simulink model "New_Traction_Control_4wheel"  (R2016a)
settings: Solver=VariableStepAuto  StartTime=0.0  StopTime=20  RelTol=1e-3
PreLoadFcn:
  | load CarSim_FE4.mat
  | load Vehicle_information_test_0118_2017.mat
libraries: fl_lib x27, nesl_utility x18, sdl_lib x8
settings Model: Creator=Ping  LastModifiedBy=Ping

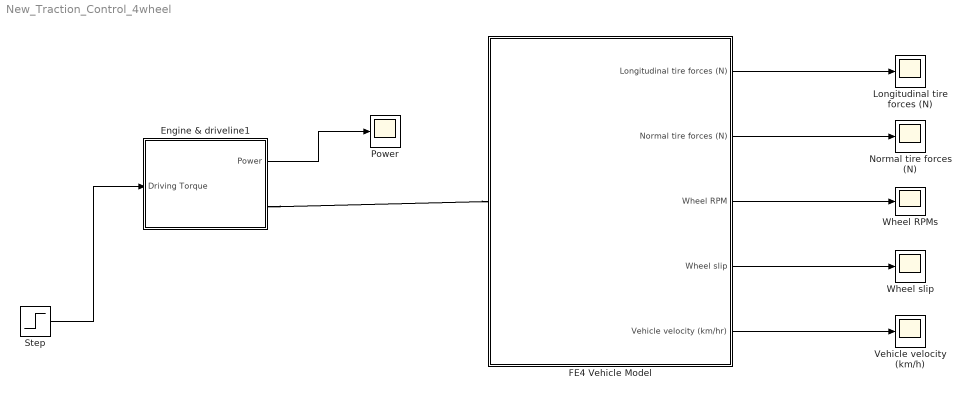
== system New_Traction_Control_4wheel ==
  Engine & driveline1 : Subsystem
  FE4 Vehicle Model : Subsystem
  Longitudinal tire forces (N) : Scope
  Normal tire forces (N) : Scope
  Power : Scope
  Step : Step  Time=10  After=500  SampleTime=0
  Vehicle velocity (km/h) : Scope
  Wheel RPMs : Scope
  Wheel slip : Scope
  wires:
  FE4 Vehicle Model/4(Wheel slip) -> Wheel slip/1
  FE4 Vehicle Model/2(Normal tire forces (N)) -> Normal tire forces (N)/1
  FE4 Vehicle Model/3(Wheel RPM) -> Wheel RPMs/1
  FE4 Vehicle Model/1(Longitudinal tire forces (N)) -> Longitudinal tire forces (N)/1
  FE4 Vehicle Model/5(Vehicle velocity (km/hr)) -> Vehicle velocity (km/h)/1
  Step/1 -> Engine & driveline1/1(Driving Torque)
  Engine & driveline1/1(Power) -> Power/1
  connections:
  Engine & driveline1/RConn1 -- FE4 Vehicle Model/LConn1

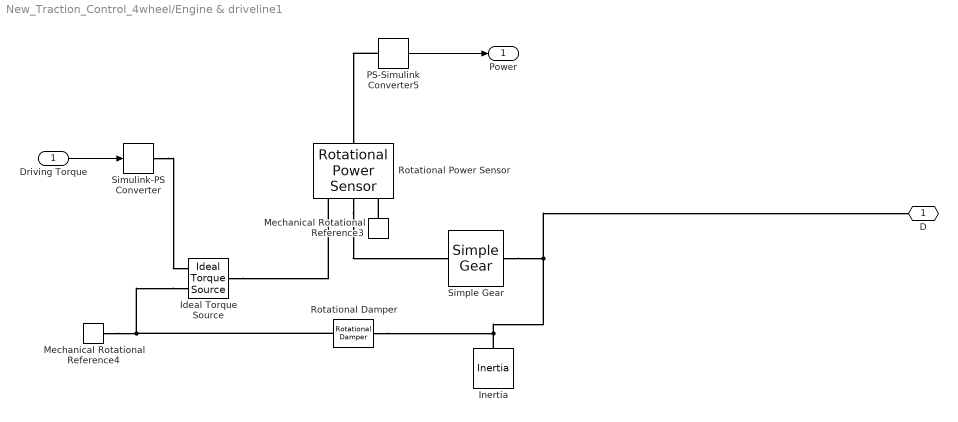
== system New_Traction_Control_4wheel/Engine & driveline1 ==
  Driving Torque : Inport
  Ideal Torque Source : fl_lib/Mechanical/Mechanical Sources/Ideal Torque Source
  Inertia : fl_lib/Mechanical/Rotational Elements/Inertia  inertia=0.015 kg*m^2  w_specify=on  w_priority=Low  w=0 rad/s  t_specify=off  t_priority=Low  t=0 N*m
  Mechanical Rotational Reference3 : fl_lib/Mechanical/Rotational Elements/Mechanical Rotational Reference
  Mechanical Rotational Reference4 : fl_lib/Mechanical/Rotational Elements/Mechanical Rotational Reference
  PS-Simulink Converter5 : nesl_utility/PS-Simulink Converter  PhysicalDomain=network_engine_domain  SubClassName=ps_output  LeftPortType=input  RightPortType=output  PseudoPeriodic=off  Frequencies=[]  Unit=kW  AffineConversion=off
  Rotational Damper : fl_lib/Mechanical/Rotational Elements/Rotational Damper  D=0.001 N*m/(rad/s)  w_specify=off  w_priority=None  w=0 rad/s  t_specify=on  t_priority=Low  t=0 N*m
  Rotational Power Sensor : sdl_lib/Sensors/Rotational Power Sensor  measurement_type=1  averaging_period=1 s  max_speed=1000 rpm  max_frequency=1000 Hz
  Simple Gear : sdl_lib/Gears/Simple Gear  ratio=4.6  rotation_direction=1  friction_model=1  T_noload=0.1 N*m  T_nom=5 N*m  efficiency_nom=0.8  efficiency=0.8  mu_visc=[ 0 0 ] N*m/(rad/s)  w_thr=0.01 rad/s  pwr_thr=0.001 W  temperature_TLU=[ 280 300 320 ] K  load_TLU=[ 1 5 10 ] N*m  efficiency_TLU=[ 0.95 0.9 0.85 ]  efficiency_TLU2=[ 0.85 0.8 0.75; 0.95 0.9 0.85; 0.85 0.8 0.7 ]  thermal_mass=50 J/K  T_init=300 K
  Simulink-PS Converter : nesl_utility/Simulink-PS Converter  PhysicalDomain=network_engine_domain  SubClassName=ps_input  LeftPortType=input  RightPortType=output  PseudoPeriodic=off  Frequencies=[]  NoiseDistribution=none  NoiseParameters=[]  Unit=N*m  AffineConversion=off  InputFiltering=off  SimscapeFilterOrder=1  InputFilterTimeConstant=0.001  UdotUserProvided=1
  D : PMIOPort  Port=1  Side=Right
  Power : Outport
  wires:
  Driving Torque/1 -> Simulink-PS Converter/1
  PS-Simulink Converter5/1 -> Power/1
  connections:
  Simple Gear/RConn1 -- D/RConn1 -- Rotational Damper/RConn1 -- Inertia/LConn1
  Ideal Torque Source/RConn2 -- Mechanical Rotational Reference4/LConn1 -- Rotational Damper/LConn1
  PS-Simulink Converter5/LConn1 -- Rotational Power Sensor/RConn1
  Mechanical Rotational Reference3/LConn1 -- Rotational Power Sensor/LConn3
  Rotational Power Sensor/LConn2 -- Simple Gear/LConn1
  Simulink-PS Converter/RConn1 -- Ideal Torque Source/RConn1
  Ideal Torque Source/LConn1 -- Rotational Power Sensor/LConn1

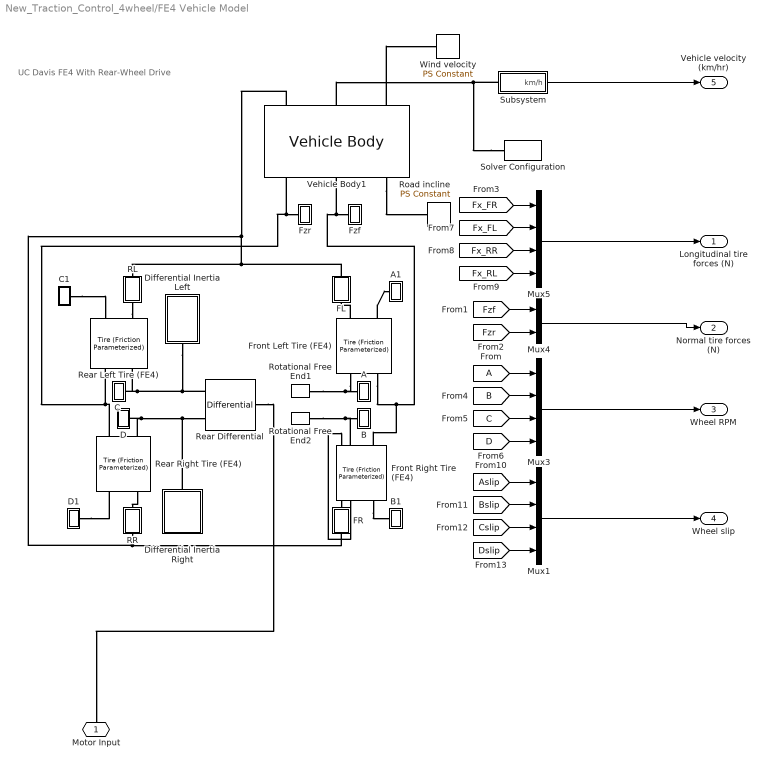
== system New_Traction_Control_4wheel/FE4 Vehicle Model ==
  note: UC Davis FE4 With Rear-Wheel Drive
  A : Subsystem
  A1 : Subsystem
  B : Subsystem
  B1 : Subsystem
  C : Subsystem
  C1 : Subsystem
  D : Subsystem
  D1 : Subsystem
  Differential Inertia Left : Subsystem
  Differential Inertia Right : Subsystem
  FL : Subsystem
  FR : Subsystem
  Front Left Tire (FE4) : sdl_lib/Tires & Vehicles/Tire (Friction Parameterized)  r_tire=r_tire m  mu_static=3  friction_model=2  mu_kinetic=0.7  slip_vector=SL  mu_kinetic_vector=Tire_nu  interp_method=2  extrap_method=1  model_compliance=0  stiffness=1e+6 N/m  damping=1000 N/(m/s)  model_inertia=1  tire_inertia=jt kg*m^2  initial_velocity=0 rad/s  model_resistance=1  resistance_model=1  coeff=0.015  p_tire=250e3 Pa  alpha=-0.003  beta=0.97  coeff_a=84e-4  coeff_b=6.2e-4 s/m  coeff_c=1.6e-4 s^2/m^2  v_thr=1e-3 m/s  v_tol=0.01 m/s  F_min=10 N  initial_traction_state=1
  Front Right Tire (FE4) : sdl_lib/Tires & Vehicles/Tire (Friction Parameterized)  r_tire=r_tire m  mu_static=3  friction_model=2  mu_kinetic=0.7  slip_vector=SL  mu_kinetic_vector=Tire_nu  interp_method=2  extrap_method=1  model_compliance=0  stiffness=1e+6 N/m  damping=1000 N/(m/s)  model_inertia=1  tire_inertia=jt kg*m^2  initial_velocity=0 rad/s  model_resistance=1  resistance_model=1  coeff=0.015  p_tire=250e3 Pa  alpha=-0.003  beta=0.97  coeff_a=84e-4  coeff_b=6.2e-4 s/m  coeff_c=1.6e-4 s^2/m^2  v_thr=1e-3 m/s  v_tol=0.01 m/s  F_min=10 N  initial_traction_state=1
  Fzf : Subsystem
  Fzr : Subsystem
  Mux1 : Mux
  Mux3 : Mux
  Mux4 : Mux  Inputs=2
  Mux5 : Mux
  RL : Subsystem
  RR : Subsystem
  Rear Differential : sdl_lib/Gears/Differential  driveshaft_location=2  cd_ratio=1  friction_model=1  efficiency=[ 0.85 0.92 ]  mu_visc=[ 0 0 ] N*m/(rad/s)  pwr_thr=[ 0.001 0.001 ] W  carrier_inertia=0 kg*m^2  planet_inertia=0 kg*m^2  temperature_TLU=[ 280 300 320 ] K  efficiency_ss_TLU=[ 0.95 0.9 0.85 ]  efficiency_cd_TLU=[ 0.95 0.9 0.85 ]  thermal_mass=50 J/K  T_init=300 K
  Rear Left Tire (FE4) : sdl_lib/Tires & Vehicles/Tire (Friction Parameterized)  r_tire=r_tire m  mu_static=3  friction_model=2  mu_kinetic=0.7  slip_vector=SL  mu_kinetic_vector=Tire_nu  interp_method=2  extrap_method=1  model_compliance=0  stiffness=1e+6 lbf/ft  damping=1000 N/(m/s)  model_inertia=1  tire_inertia=jt kg*m^2  initial_velocity=0 rad/s  model_resistance=1  resistance_model=1  coeff=0.015  p_tire=250e3 Pa  alpha=-0.003  beta=0.97  coeff_a=84e-4  coeff_b=6.2e-4 s/m  coeff_c=1.6e-4 s^2/m^2  v_thr=1e-3 m/s  v_tol=0.01 m/s  F_min=10 N  initial_traction_state=1
  Rear Right Tire (FE4) : sdl_lib/Tires & Vehicles/Tire (Friction Parameterized)  r_tire=r_tire m  mu_static=3  friction_model=2  mu_kinetic=0.7  slip_vector=SL  mu_kinetic_vector=Tire_nu  interp_method=2  extrap_method=1  model_compliance=0  stiffness=1e+6 lbf/ft  damping=1000 N/(m/s)  model_inertia=1  tire_inertia=jt kg*m^2  initial_velocity=0 rad/s  model_resistance=1  resistance_model=1  coeff=0.015  p_tire=250e3 Pa  alpha=-0.003  beta=0.97  coeff_a=84e-4  coeff_b=6.2e-4 s/m  coeff_c=1.6e-4 s^2/m^2  v_thr=1e-3 m/s  v_tol=0.01 m/s  F_min=10 N  initial_traction_state=1
  Road incline : fl_lib/Physical Signals/Sources/PS Constant  constant=0
  Rotational Free End1 : fl_lib/Mechanical/Rotational Elements/Rotational Free End  w_specify=on  w_priority=Low  w=0 rad/s
  Rotational Free End2 : fl_lib/Mechanical/Rotational Elements/Rotational Free End  w_specify=on  w_priority=Low  w=0 rad/s
  Solver Configuration : nesl_utility/Solver Configuration  PhysicalDomain=network_engine_domain  SubClassName=solver  LeftPortType=input  RightPortType=generic  Accelerate=off  Tones=[]  Harmonics=[]  SimulateNoise=off  Profile=off  UseLocalSampling=off  EnableSwitchedLinearOptims=on  FrequencyDomain=off  UseCCode=off  RelTol=0.001  AbsTol=1e-06  MinStep=1e-09  ToWorkspace=off  RevertToSquareIcSolve=off  NumHomotopyIterations=100  PhasorMode=off  PhasorModeNumHarmonics=1  OverrideAbsTol=off  DoDC=off  ResidualTolerance=1e-9  UseLocalSolver=off  LocalSolverChoice=NE_BACKWARD_EULER_ADVANCER  LocalSolverSampleTime=0.1  DoFixedCost=off  MaxNonlinIter=3  MaxModeIter=2  LinearAlgebra=Sparse  DelaysMemoryBudget=1024  AutomaticFiltering=on  FilteringTimeConstant=0.001
  Subsystem : Subsystem
  Vehicle Body1 : sdl_lib/Tires & Vehicles/Vehicle Body  mass=m_total kg  n_w=2  x_f=aa m  x_r=bb m  y_c=hf m  area=frontal_area m^2  Cd=Cd  v0=0 m/s
  Wind velocity : fl_lib/Physical Signals/Sources/PS Constant  constant=0
  Motor Input : PMIOPort  Port=1  Side=Left
  Longitudinal tire forces (N) : Outport
  Normal tire forces (N) : Outport  Port=2
  Wheel RPM : Outport  Port=3
  Wheel slip : Outport  Port=4
  Vehicle velocity (km/hr) : Outport  Port=5
  wires:
  Subsystem/1(km/h) -> Vehicle velocity (km/hr)/1
  [A] -> Mux3/1
  [Fx_FL] -> Mux5/2
  [Fx_FR] -> Mux5/1
  [Fx_RR] -> Mux5/3
  [Fx_RL] -> Mux5/4
  [Aslip] -> Mux1/1
  [Dslip] -> Mux1/4
  Mux1/1 -> Wheel slip/1
  [Bslip] -> Mux1/2
  [Fzr] -> Mux4/2
  Mux4/1 -> Normal tire forces (N)/1
  [Cslip] -> Mux1/3
  [C] -> Mux3/3
  [B] -> Mux3/2
  [D] -> Mux3/4
  Mux3/1 -> Wheel RPM/1
  [Fzf] -> Mux4/1
  Mux5/1 -> Longitudinal tire forces (N)/1
  connections:
  C1/LConn1 -- Rear Left Tire (FE4)/RConn1
  Rear Right Tire (FE4)/RConn2 -- RR/LConn1
  Rotational Free End2/LConn1 -- Front Right Tire (FE4)/LConn2 -- B/LConn1
  A/LConn1 -- Rotational Free End1/LConn1 -- Front Left Tire (FE4)/LConn2
  Rear Differential/LConn1 -- Motor Input/RConn1
  Front Right Tire (FE4)/RConn1 -- B1/LConn1
  Vehicle Body1/LConn3 -- Wind velocity/RConn1
  D1/LConn1 -- Rear Right Tire (FE4)/RConn1
  Front Left Tire (FE4)/RConn1 -- A1/LConn1
  RR/RConn1 -- FR/RConn1 -- Vehicle Body1/LConn1 -- FL/RConn1 -- RL/RConn1
  D/LConn1 -- Rear Right Tire (FE4)/LConn2 -- Differential Inertia Right/RConn1 -- Rear Differential/RConn2
  Fzr/LConn1 -- Rear Right Tire (FE4)/LConn1 -- Rear Left Tire (FE4)/LConn1 -- Vehicle Body1/RConn1
  Solver Configuration/RConn1 -- Vehicle Body1/LConn2 -- Subsystem/LConn1
  Fzf/LConn1 -- Front Left Tire (FE4)/LConn1 -- Front Right Tire (FE4)/LConn1 -- Vehicle Body1/RConn2
  Vehicle Body1/RConn3 -- Road incline/RConn1
  RL/LConn1 -- Rear Left Tire (FE4)/RConn2
  Front Right Tire (FE4)/RConn2 -- FR/LConn1
  Front Left Tire (FE4)/RConn2 -- FL/LConn1
  Rear Differential/RConn1 -- C/LConn1 -- Rear Left Tire (FE4)/LConn2 -- Differential Inertia Left/RConn1

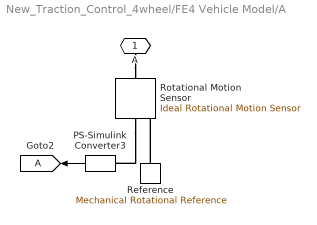
== system New_Traction_Control_4wheel/FE4 Vehicle Model/A ==
  PS-Simulink Converter3 : nesl_utility/PS-Simulink Converter  PhysicalDomain=network_engine_domain  SubClassName=ps_output  LeftPortType=input  RightPortType=output  PseudoPeriodic=off  Frequencies=[]  Unit=rpm  AffineConversion=off
  Reference : fl_lib/Mechanical/Rotational Elements/Mechanical Rotational Reference
  Rotational Motion Sensor : fl_lib/Mechanical/Mechanical Sensors/Ideal Rotational Motion Sensor  offset=0 rad
  A : PMIOPort  Port=1  Side=Left
  tag scope: A=global
  wires:
  PS-Simulink Converter3/1 -> [A]
  connections:
  Rotational Motion Sensor/RConn2 -- PS-Simulink Converter3/LConn1
  Reference/LConn1 -- Rotational Motion Sensor/RConn1
  A/RConn1 -- Rotational Motion Sensor/LConn1

== system New_Traction_Control_4wheel/FE4 Vehicle Model/A1 ==
  PS-Simulink Converter : nesl_utility/PS-Simulink Converter  PhysicalDomain=network_engine_domain  SubClassName=ps_output  LeftPortType=input  RightPortType=output  PseudoPeriodic=off  Frequencies=[]  Unit=1  AffineConversion=off
  S : PMIOPort  Port=1  Side=Left
  tag scope: Aslip=global
  wires:
  PS-Simulink Converter/1 -> [Aslip]
  connections:
  S/RConn1 -- PS-Simulink Converter/LConn1

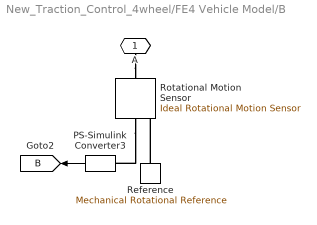
== system New_Traction_Control_4wheel/FE4 Vehicle Model/B ==
  PS-Simulink Converter3 : nesl_utility/PS-Simulink Converter  PhysicalDomain=network_engine_domain  SubClassName=ps_output  LeftPortType=input  RightPortType=output  PseudoPeriodic=off  Frequencies=[]  Unit=rpm  AffineConversion=off
  Reference : fl_lib/Mechanical/Rotational Elements/Mechanical Rotational Reference
  Rotational Motion Sensor : fl_lib/Mechanical/Mechanical Sensors/Ideal Rotational Motion Sensor  offset=0 rad
  A : PMIOPort  Port=1  Side=Left
  tag scope: B=global
  wires:
  PS-Simulink Converter3/1 -> [B]
  connections:
  A/RConn1 -- Rotational Motion Sensor/LConn1
  Reference/LConn1 -- Rotational Motion Sensor/RConn1
  Rotational Motion Sensor/RConn2 -- PS-Simulink Converter3/LConn1

== system New_Traction_Control_4wheel/FE4 Vehicle Model/B1 ==
  PS-Simulink Converter : nesl_utility/PS-Simulink Converter  PhysicalDomain=network_engine_domain  SubClassName=ps_output  LeftPortType=input  RightPortType=output  PseudoPeriodic=off  Frequencies=[]  Unit=1  AffineConversion=off
  S : PMIOPort  Port=1  Side=Left
  tag scope: Bslip=global
  wires:
  PS-Simulink Converter/1 -> [Bslip]
  connections:
  S/RConn1 -- PS-Simulink Converter/LConn1

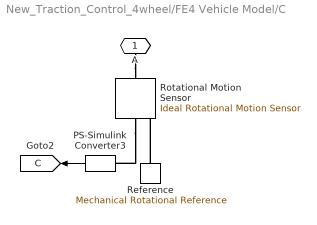
== system New_Traction_Control_4wheel/FE4 Vehicle Model/C ==
  PS-Simulink Converter3 : nesl_utility/PS-Simulink Converter  PhysicalDomain=network_engine_domain  SubClassName=ps_output  LeftPortType=input  RightPortType=output  PseudoPeriodic=off  Frequencies=[]  Unit=rpm  AffineConversion=off
  Reference : fl_lib/Mechanical/Rotational Elements/Mechanical Rotational Reference
  Rotational Motion Sensor : fl_lib/Mechanical/Mechanical Sensors/Ideal Rotational Motion Sensor  offset=0 rad
  A : PMIOPort  Port=1  Side=Left
  tag scope: C=global
  wires:
  PS-Simulink Converter3/1 -> [C]
  connections:
  Rotational Motion Sensor/RConn2 -- PS-Simulink Converter3/LConn1
  Reference/LConn1 -- Rotational Motion Sensor/RConn1
  A/RConn1 -- Rotational Motion Sensor/LConn1

== system New_Traction_Control_4wheel/FE4 Vehicle Model/C1 ==
  PS-Simulink Converter : nesl_utility/PS-Simulink Converter  PhysicalDomain=network_engine_domain  SubClassName=ps_output  LeftPortType=input  RightPortType=output  PseudoPeriodic=off  Frequencies=[]  Unit=1  AffineConversion=off
  S : PMIOPort  Port=1  Side=Left
  tag scope: Cslip=global
  wires:
  PS-Simulink Converter/1 -> [Cslip]
  connections:
  S/RConn1 -- PS-Simulink Converter/LConn1

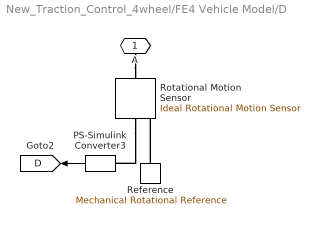
== system New_Traction_Control_4wheel/FE4 Vehicle Model/D ==
  PS-Simulink Converter3 : nesl_utility/PS-Simulink Converter  PhysicalDomain=network_engine_domain  SubClassName=ps_output  LeftPortType=input  RightPortType=output  PseudoPeriodic=off  Frequencies=[]  Unit=rpm  AffineConversion=off
  Reference : fl_lib/Mechanical/Rotational Elements/Mechanical Rotational Reference
  Rotational Motion Sensor : fl_lib/Mechanical/Mechanical Sensors/Ideal Rotational Motion Sensor  offset=0 rad
  A : PMIOPort  Port=1  Side=Left
  tag scope: D=global
  wires:
  PS-Simulink Converter3/1 -> [D]
  connections:
  A/RConn1 -- Rotational Motion Sensor/LConn1
  Reference/LConn1 -- Rotational Motion Sensor/RConn1
  Rotational Motion Sensor/RConn2 -- PS-Simulink Converter3/LConn1

== system New_Traction_Control_4wheel/FE4 Vehicle Model/D1 ==
  PS-Simulink Converter : nesl_utility/PS-Simulink Converter  PhysicalDomain=network_engine_domain  SubClassName=ps_output  LeftPortType=input  RightPortType=output  PseudoPeriodic=off  Frequencies=[]  Unit=1  AffineConversion=off
  S : PMIOPort  Port=1  Side=Left
  tag scope: Dslip=global
  wires:
  PS-Simulink Converter/1 -> [Dslip]
  connections:
  S/RConn1 -- PS-Simulink Converter/LConn1

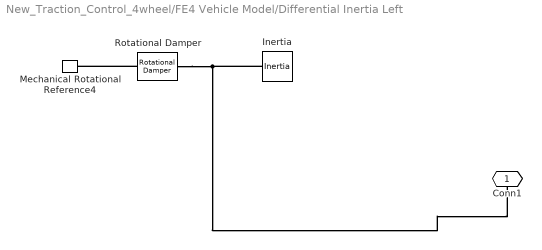
== system New_Traction_Control_4wheel/FE4 Vehicle Model/Differential Inertia Left ==
  Inertia : fl_lib/Mechanical/Rotational Elements/Inertia  inertia=0.015 kg*m^2  w_specify=on  w_priority=Low  w=0 rad/s  t_specify=off  t_priority=Low  t=0 N*m
  Mechanical Rotational Reference4 : fl_lib/Mechanical/Rotational Elements/Mechanical Rotational Reference
  Rotational Damper : fl_lib/Mechanical/Rotational Elements/Rotational Damper  D=0.001 N*m/(rad/s)  w_specify=off  w_priority=None  w=0 rad/s  t_specify=on  t_priority=Low  t=0 N*m
  Conn1 : PMIOPort  Port=1  Side=Right
  connections:
  Rotational Damper/RConn1 -- Conn1/RConn1 -- Inertia/LConn1
  Rotational Damper/LConn1 -- Mechanical Rotational Reference4/LConn1

== system New_Traction_Control_4wheel/FE4 Vehicle Model/Differential Inertia Right ==
  Inertia : fl_lib/Mechanical/Rotational Elements/Inertia  inertia=0.015 kg*m^2  w_specify=on  w_priority=Low  w=0 rad/s  t_specify=off  t_priority=Low  t=0 N*m
  Mechanical Rotational Reference4 : fl_lib/Mechanical/Rotational Elements/Mechanical Rotational Reference
  Rotational Damper : fl_lib/Mechanical/Rotational Elements/Rotational Damper  D=0.001 N*m/(rad/s)  w_specify=off  w_priority=None  w=0 rad/s  t_specify=on  t_priority=Low  t=0 N*m
  Conn1 : PMIOPort  Port=1  Side=Right
  connections:
  Rotational Damper/LConn1 -- Mechanical Rotational Reference4/LConn1
  Conn1/RConn1 -- Inertia/LConn1 -- Rotational Damper/RConn1

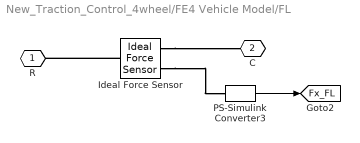
== system New_Traction_Control_4wheel/FE4 Vehicle Model/FL ==
  Ideal Force Sensor : fl_lib/Mechanical/Mechanical Sensors/Ideal Force Sensor
  PS-Simulink Converter3 : nesl_utility/PS-Simulink Converter  PhysicalDomain=network_engine_domain  SubClassName=ps_output  LeftPortType=input  RightPortType=output  PseudoPeriodic=off  Frequencies=[]  Unit=N  AffineConversion=off
  R : PMIOPort  Port=1  Side=Left
  C : PMIOPort  Port=2  Side=Right
  tag scope: Fx_FL=global
  wires:
  PS-Simulink Converter3/1 -> [Fx_FL]
  connections:
  Ideal Force Sensor/LConn1 -- R/RConn1
  Ideal Force Sensor/RConn1 -- C/RConn1
  Ideal Force Sensor/RConn2 -- PS-Simulink Converter3/LConn1

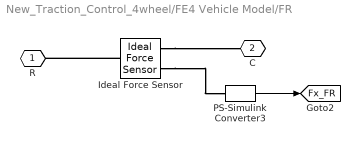
== system New_Traction_Control_4wheel/FE4 Vehicle Model/FR ==
  Ideal Force Sensor : fl_lib/Mechanical/Mechanical Sensors/Ideal Force Sensor
  PS-Simulink Converter3 : nesl_utility/PS-Simulink Converter  PhysicalDomain=network_engine_domain  SubClassName=ps_output  LeftPortType=input  RightPortType=output  PseudoPeriodic=off  Frequencies=[]  Unit=N  AffineConversion=off
  R : PMIOPort  Port=1  Side=Left
  C : PMIOPort  Port=2  Side=Right
  tag scope: Fx_FR=global
  wires:
  PS-Simulink Converter3/1 -> [Fx_FR]
  connections:
  Ideal Force Sensor/RConn2 -- PS-Simulink Converter3/LConn1
  Ideal Force Sensor/RConn1 -- C/RConn1
  Ideal Force Sensor/LConn1 -- R/RConn1

== system New_Traction_Control_4wheel/FE4 Vehicle Model/Fzf ==
  PS-Simulink Converter3 : nesl_utility/PS-Simulink Converter  PhysicalDomain=network_engine_domain  SubClassName=ps_output  LeftPortType=input  RightPortType=output  PseudoPeriodic=off  Frequencies=[]  Unit=N  AffineConversion=off
  f : PMIOPort  Port=1  Side=Left
  tag scope: Fzf=global
  wires:
  PS-Simulink Converter3/1 -> [Fzf]
  connections:
  f/RConn1 -- PS-Simulink Converter3/LConn1

== system New_Traction_Control_4wheel/FE4 Vehicle Model/Fzr ==
  PS-Simulink Converter3 : nesl_utility/PS-Simulink Converter  PhysicalDomain=network_engine_domain  SubClassName=ps_output  LeftPortType=input  RightPortType=output  PseudoPeriodic=off  Frequencies=[]  Unit=N  AffineConversion=off
  f : PMIOPort  Port=1  Side=Left
  tag scope: Fzr=global
  wires:
  PS-Simulink Converter3/1 -> [Fzr]
  connections:
  f/RConn1 -- PS-Simulink Converter3/LConn1

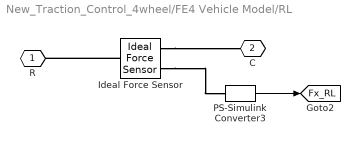
== system New_Traction_Control_4wheel/FE4 Vehicle Model/RL ==
  Ideal Force Sensor : fl_lib/Mechanical/Mechanical Sensors/Ideal Force Sensor
  PS-Simulink Converter3 : nesl_utility/PS-Simulink Converter  PhysicalDomain=network_engine_domain  SubClassName=ps_output  LeftPortType=input  RightPortType=output  PseudoPeriodic=off  Frequencies=[]  Unit=N  AffineConversion=off
  R : PMIOPort  Port=1  Side=Left
  C : PMIOPort  Port=2  Side=Right
  tag scope: Fx_RL=global
  wires:
  PS-Simulink Converter3/1 -> [Fx_RL]
  connections:
  Ideal Force Sensor/RConn2 -- PS-Simulink Converter3/LConn1
  Ideal Force Sensor/RConn1 -- C/RConn1
  Ideal Force Sensor/LConn1 -- R/RConn1

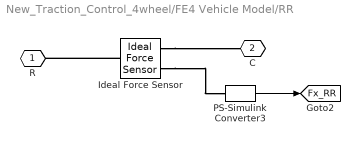
== system New_Traction_Control_4wheel/FE4 Vehicle Model/RR ==
  Ideal Force Sensor : fl_lib/Mechanical/Mechanical Sensors/Ideal Force Sensor
  PS-Simulink Converter3 : nesl_utility/PS-Simulink Converter  PhysicalDomain=network_engine_domain  SubClassName=ps_output  LeftPortType=input  RightPortType=output  PseudoPeriodic=off  Frequencies=[]  Unit=N  AffineConversion=off
  R : PMIOPort  Port=1  Side=Left
  C : PMIOPort  Port=2  Side=Right
  tag scope: Fx_RR=global
  wires:
  PS-Simulink Converter3/1 -> [Fx_RR]
  connections:
  Ideal Force Sensor/LConn1 -- R/RConn1
  Ideal Force Sensor/RConn1 -- C/RConn1
  Ideal Force Sensor/RConn2 -- PS-Simulink Converter3/LConn1

== system New_Traction_Control_4wheel/FE4 Vehicle Model/Subsystem ==
  PS-Simulink Converter1 : nesl_utility/PS-Simulink Converter  PhysicalDomain=network_engine_domain  SubClassName=ps_output  LeftPortType=input  RightPortType=output  PseudoPeriodic=off  Frequencies=[]  Unit=m/s  AffineConversion=off
  m/s2km/h : Gain  Gain=60*60/1000
  V : PMIOPort  Port=1  Side=Left
  km/h : Outport
  wires:
  PS-Simulink Converter1/1 -> m/s2km/h/1
  m/s2km/h/1 -> km/h/1
  connections:
  V/RConn1 -- PS-Simulink Converter1/LConn1
